simulink model "ExampleQueryPoints"  (Simulink 9.2)
settings: Solver=FixedStepDiscrete  StartTime=0.0  StopTime=inf  FixedStep=0.001  MaxStep=0.01  RelTol=1e-3  EnableMultiTasking=on
libraries: rFproPhysicsLib x5
settings Model: Creator=enewton  LastModifiedBy=SeanKavanagh
settings OptimizationCC: ExpressionDepthLimit=2147483647
settings DebuggingCC: SolverPrmCheckMsg=warning
settings HardwareCC: TargetBitPerPointer=64  TargetBitPerSizeT=64  TargetBitPerPtrDiffT=64  TargetLongLongMode=on  TargetIntDivRoundTo=Zero  TargetEndianess=LittleEndian  TargetWordSize=64  TargetHWDeviceType=MATLAB Host  ProdEqTarget=off
settings RTWCC: SystemTargetFile=rsim.tlc  TemplateMakefile=rsim_default_tmf  Description=Rapid Simulation Target  TargetLang=C++
settings RSimTargetCC: PreserveStateflowLocalDataDimensions=off

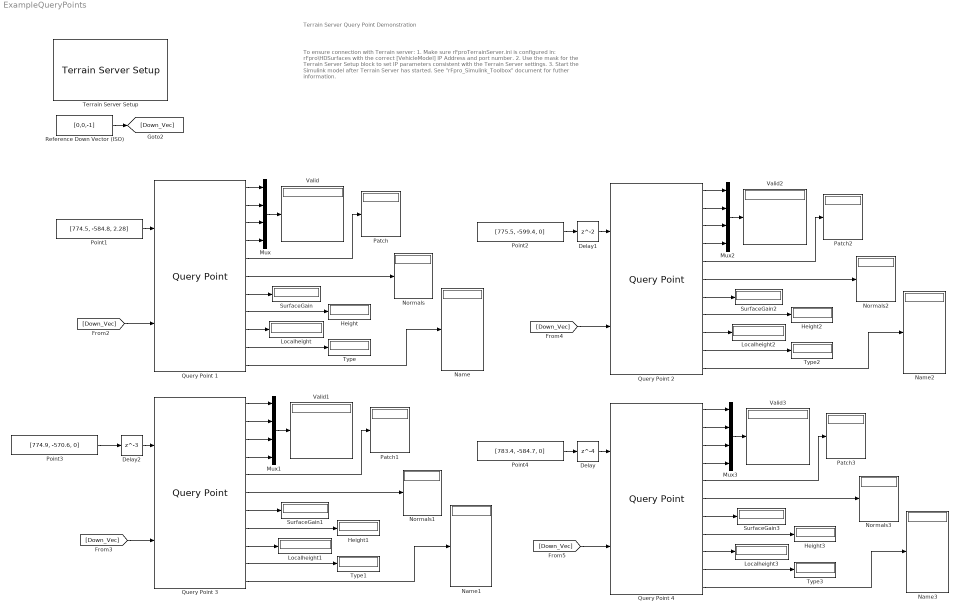
== system ExampleQueryPoints ==
  note: Terrain Server Query Point Demonstration
  note: To ensure connection with Terrain server:
      |
      | 1. Make sure rFproTerrainServer.ini is configured in: rFpro\HDSurfaces with the correct
      |     [VehicleModel] IP Address and port number.
      |
      | 2. Use the mask for the Terrain Server Setup block to set IP parameters consistent with
      |     the Terrain Server settings.
      |
      | 3. Start the Simulink model after Terrain Server has started.
      |
      | See "rFpro_Simulink_Toolbox" document for futher information.
  Delay : Delay  DelayLength=4
  Delay1 : Delay
  Delay2 : Delay  DelayLength=3
  Height{,1..3} (4 alike) : Display
  Localheight{,1..3} (4 alike) : Display
  Mux{,1..3} (4 alike) : Mux
  Name{,1..3} (4 alike) : Display
  Normals{,1..3} (4 alike) : Display
  Patch{,1..3} (4 alike) : Display
  Point1 : Constant  Value=[774.5, -584.8, 2.28]  VectorParams1D=off
  Point2 : Constant  Value=[775.5, -599.4, 0]  VectorParams1D=off
  Point3 : Constant  Value=[774.9, -570.6, 0]  VectorParams1D=off
  Point4 : Constant  Value=[783.4, -584.7, 0]  VectorParams1D=off
  Query Point 1 : rFproPhysicsLib/Terrain Server Blocks/Query Point  iso_mode=on  queryID_start=1  queryID_step=4  useReverseByteOrder=off  rFpro__TS_platform=Remote Model - Default
  Query Point 2 : rFproPhysicsLib/Terrain Server Blocks/Query Point  iso_mode=on  queryID_start=2  queryID_step=4  useReverseByteOrder=off  rFpro__TS_platform=Remote Model - Default
  Query Point 3 : rFproPhysicsLib/Terrain Server Blocks/Query Point  iso_mode=on  queryID_start=3  queryID_step=4  useReverseByteOrder=off  rFpro__TS_platform=Remote Model - Default
  Query Point 4 : rFproPhysicsLib/Terrain Server Blocks/Query Point  iso_mode=on  queryID_start=4  queryID_step=4  useReverseByteOrder=off  rFpro__TS_platform=Remote Model - Default
  Reference Down Vector (ISO) : Constant  Value=[0,0,-1]
  SurfaceGain{,1..3} (4 alike) : Display
  Terrain Server Setup : rFproPhysicsLib/Terrain Server Blocks/Terrain Server Setup  Priority=0  track_name=''  tyre_config=[]  points_config=[]  iso=on  triggerOnHeartbeat=off  heartbeat_latency=1750  rFpro__platform=Remote Model - Default  ts_address='127.0.0.1'  ts_port=11006  sendSampleTime=-1  sl_address='127.0.0.1'  sl_port=11002  receiveSampleTime=-1  maxUDPMsgs=2  useReverseByteOrder=off
  Type{,1..3} (4 alike) : Display
  Valid{,1..3} (4 alike) : Display
  wires:
  Query Point 1/9 -> Localheight/1
  Query Point 1/8 -> Height/1
  Query Point 1/7 -> SurfaceGain/1
  Query Point 1/6 -> Normals/1
  Mux/1 -> Valid/1
  Query Point 1/11 -> Name/1
  Query Point 1/10 -> Type/1
  Query Point 1/4 -> Mux/4
  Query Point 1/1 -> Mux/1
  Query Point 1/3 -> Mux/3
  Query Point 1/2 -> Mux/2
  Query Point 1/5 -> Patch/1
  Point2/1 -> Delay1/1
  Point3/1 -> Delay2/1
  Point4/1 -> Delay/1
  Query Point 3/9 -> Localheight1/1
  Query Point 3/8 -> Height1/1
  Query Point 3/7 -> SurfaceGain1/1
  Query Point 3/6 -> Normals1/1
  Mux1/1 -> Valid1/1
  Query Point 3/11 -> Name1/1
  Query Point 3/10 -> Type1/1
  Query Point 3/4 -> Mux1/4
  Query Point 3/1 -> Mux1/1
  Query Point 3/3 -> Mux1/3
  Query Point 3/2 -> Mux1/2
  Query Point 3/5 -> Patch1/1
  Query Point 2/9 -> Localheight2/1
  Query Point 2/8 -> Height2/1
  Query Point 2/7 -> SurfaceGain2/1
  Query Point 2/6 -> Normals2/1
  Mux2/1 -> Valid2/1
  Query Point 2/11 -> Name2/1
  Query Point 2/10 -> Type2/1
  Query Point 2/5 -> Patch2/1
  Query Point 2/4 -> Mux2/4
  Query Point 2/2 -> Mux2/2
  Query Point 2/1 -> Mux2/1
  Query Point 2/3 -> Mux2/3
  Query Point 4/9 -> Localheight3/1
  Query Point 4/8 -> Height3/1
  Query Point 4/7 -> SurfaceGain3/1
  Query Point 4/6 -> Normals3/1
  Mux3/1 -> Valid3/1
  Query Point 4/11 -> Name3/1
  Query Point 4/10 -> Type3/1
  Query Point 4/5 -> Patch3/1
  Query Point 4/4 -> Mux3/4
  Query Point 4/2 -> Mux3/2
  Query Point 4/1 -> Mux3/1
  Query Point 4/3 -> Mux3/3
  Reference Down Vector (ISO)/1 -> [Down_Vec]
  [Down_Vec] -> Query Point 1/2
  [Down_Vec] -> Query Point 3/2
  [Down_Vec] -> Query Point 4/2
  [Down_Vec] -> Query Point 2/2
  Point1/1 -> Query Point 1/1
  Delay2/1 -> Query Point 3/1
  Delay1/1 -> Query Point 2/1
  Delay/1 -> Query Point 4/1
